simulink model "SimModel_R2019a_RL"  (R2019a)
settings: Solver=ode5  StartTime=0.0  StopTime=120  FixedStep=dt  RelTol=1e-3  EnableMultiTasking=on
values from neighbouring files (symbols this model uses):
  D_a1 = 0.1000    (= 0.1)    [SimModel_R2019a_RL_Para.m]
  D_a2 = 0.0500    (= 0.05)    [SimModel_R2019a_RL_Para.m]
  D_a3 = 3.7000    (= 3.7)    [SimModel_R2019a_RL_Para.m]
  D_a4 = 0.0    (= 0)    [SimModel_R2019a_RL_Para.m]
  D_K2 = 1.0*1.00    (= 1)    [SimModel_R2019a_RL_Para.m]
  D_Knms = 1.0    (= 1)    [SimModel_R2019a_RL_Para.m]
  D_TFar = 1.0    (= 1)    [SimModel_R2019a_RL_Para.m]
  D_Tn = 0.1000    (= 0.1)    [SimModel_R2019a_RL_Para.m]
  D_TNear = 0.3    [SimModel_R2019a_RL_Para.m]
  Et = 0.026    [SimModel_R2019a_RL_Para.m]
  Gain_EA_Far = 0    [SimModel_R2019a_RL_Para.m]
  H_a1 = 2.000    (= 2)    [SimModel_R2019a_RL_Para.m]
  H_a2 = 0.0500    (= 0.05)    [SimModel_R2019a_RL_Para.m]
  H_a3 = 40.0    (= 40)    [SimModel_R2019a_RL_Para.m]
  H_a4 = 1.0    (= 1)    [SimModel_R2019a_RL_Para.m]
  H_TFar = 0.7    [SimModel_R2019a_RL_Para.m]
  H_TNear = 0.3    [SimModel_R2019a_RL_Para.m]
  I = 300*9.8    (= 2940)    [SimModel_R2019a_RL_Para.m]
  Ih = 0.11    [SimModel_R2019a_RL_Para.m]
  K1 = 1    [SimModel_R2019a_RL_Para.m]
  Kda = 0.57    [SimModel_R2019a_RL_Para.m]
  Kf = 5.33e+04    (= 53300)    [SimModel_R2019a_RL_Para.m]
  Kr = 1.17e+05    (= 117000)    [SimModel_R2019a_RL_Para.m]
  Ks = 4950*9.8    (= 48510)    [SimModel_R2019a_RL_Para.m]
  Ksa = 0.0    (= 0)    [SimModel_R2019a_RL_Para.m]
  Kt = 1/17    (= 0.0588235294118)    [SimModel_R2019a_RL_Para.m]
  lf = 1.00    (= 1)    [SimModel_R2019a_RL_Para.m]
  lr = 1.635    [SimModel_R2019a_RL_Para.m]
  m = 1100    [SimModel_R2019a_RL_Para.m]
  TT = csvread('XY_TT.csv',0,1)    [SimModel_R2019a_RL_Para.m]
  V = 60/3.6    (= 16.6666666667)    [SimModel_R2019a_RL_Para.m]
undefined symbols (not defined in the file or in its folder): Band_TH, D_KHG, D_Kw, D_Td, dt, H_K2, Random_Disturbance
libraries: simulink x3, rllib x1
settings Model: ModifiedByFormat=kelejichi  Creator=kelejichi  LastModifiedBy=kelejichi
settings DataIOCC: SaveFormat=Array  SignalLoggingSaveFormat=ModelDataLogs
settings OptimizationCC: ExpressionDepthLimit=2147483647  InitFltsAndDblsToZero=on  LifeSpan=inf
settings DebuggingCC: UnderspecifiedInitializationDetection=Classic  MergeDetectMultiDrivingBlocksExec=none  SolverPrmCheckMsg=warning  FcnCallInpInsideContextMsg=warning  AllowSymbolicDim=off  StateNameClashWarn=warning  SFUnexpectedBacktrackingDiag=warning  SFNoUnconditionalDefaultTransitionDiag=warning  SFExecutionAtInitializationDiag=none  ArithmeticOperatorsInVariantConditions=warning
settings HardwareCC: ProdBitPerPointer=32  ProdBitPerSizeT=32  ProdBitPerPtrDiffT=32  ProdLargestAtomicFloat=None  ProdIntDivRoundTo=Undefined  ProdEndianess=Unspecified  ProdWordSize=32  ProdHWDeviceType=32-bit Generic
settings ModelReferenceCC: PropagateSignalLabelsOutOfModel=off
settings SFSimCC: SimUseLocalCustomCode=off
settings RTWCC: RTWUseLocalCustomCode=off
settings CodeAppCC: StateflowObjectComments=on
settings GRTTargetCC: TargetLangStandard=C89/C90 (ANSI)  GeneratePreprocessorConditionals=Disable all  CombineOutputUpdateFcns=off  GRTInterface=on
settings ConfigComp: CovMetricSettings=dw  CovHtmlReporting=on  CovSaveCumulativeToWorkspaceVar=on  CovSaveSingleToWorkspaceVar=on  CovExternalEMLEnable=off

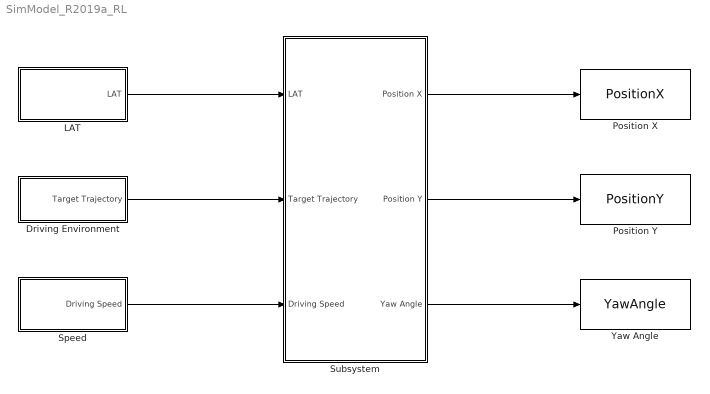
== system SimModel_R2019a_RL ==
  Driving Environment : Subsystem
  LAT : Subsystem
  Position X : ToWorkspace  VariableName=PositionX  SaveFormat=Timeseries  SampleTime=-1
  Position Y : ToWorkspace  VariableName=PositionY  SaveFormat=Timeseries  SampleTime=-1
  Speed : Subsystem
  Subsystem : Subsystem
  Yaw Angle : ToWorkspace  VariableName=YawAngle  SaveFormat=Timeseries  SampleTime=-1
  wires:
  Speed/1(Driving Speed) -> Subsystem/3(Driving Speed)
  Driving Environment/1(Target Trajectory) -> Subsystem/2(Target Trajectory)
  Subsystem/1(Position X) -> Position X/1
  Subsystem/2(Position Y) -> Position Y/1
  Subsystem/3(Yaw Angle) -> Yaw Angle/1
  LAT/1(LAT) -> Subsystem/1(LAT)

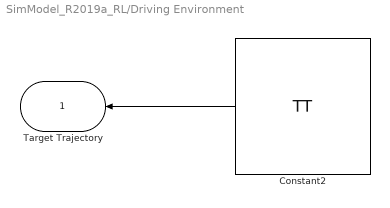
== system SimModel_R2019a_RL/Driving Environment ==
  Constant2 : Constant  Value=TT
  Target Trajectory : Outport
  wires:
  Constant2/1 -> Target Trajectory/1

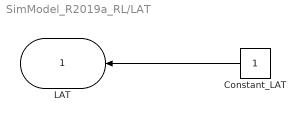
== system SimModel_R2019a_RL/LAT ==
  Constant_LAT : Constant
  LAT : Outport
  wires:
  Constant_LAT/1 -> LAT/1

== system SimModel_R2019a_RL/Speed ==
  Constant1 : Constant  Value=V
  Driving Speed : Outport
  wires:
  Constant1/1 -> Driving Speed/1

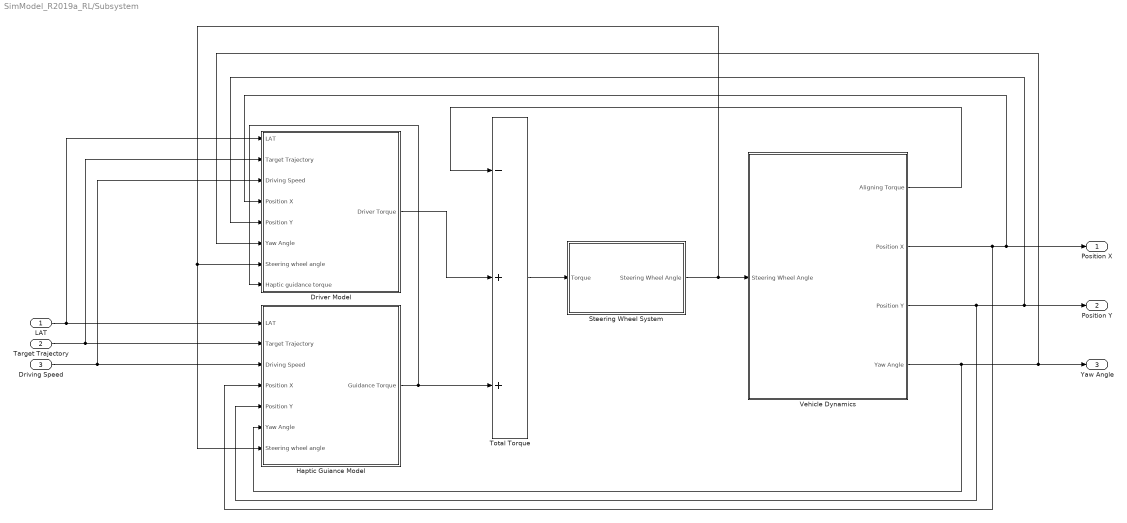
== system SimModel_R2019a_RL/Subsystem ==
  LAT : Inport
  Target Trajectory : Inport  Port=2
  Driving Speed : Inport  Port=3
  Driver Model : Subsystem
  Haptic Guiance Model : Subsystem
  Steering Wheel System : Subsystem
  Total Torque : Sum  Inputs=-++
  Vehicle Dynamics : Subsystem
  Position X : Outport
  Position Y : Outport  Port=2
  Yaw Angle : Outport  Port=3
  wires:
  Vehicle Dynamics/1(Aligning Torque) -> Total Torque/1
  Vehicle Dynamics/2(Position X) -> Position X/1, Driver Model/4(Position X), Haptic Guiance Model/4(Position X)
  Total Torque/1 -> Steering Wheel System/1(Torque)
  Driving Speed/1 -> Haptic Guiance Model/3(Driving Speed), Driver Model/3(Driving Speed)
  Target Trajectory/1 -> Driver Model/2(Target Trajectory), Haptic Guiance Model/2(Target Trajectory)
  Haptic Guiance Model/1(Guidance Torque) -> Total Torque/3, Driver Model/8(Haptic guidance torque)
  Vehicle Dynamics/3(Position Y) -> Position Y/1, Driver Model/5(Position Y), Haptic Guiance Model/5(Position Y)
  Vehicle Dynamics/4(Yaw Angle) -> Yaw Angle/1, Driver Model/6(Yaw Angle), Haptic Guiance Model/6(Yaw Angle)
  Driver Model/1(Driver Torque) -> Total Torque/2
  LAT/1 -> Driver Model/1(LAT), Haptic Guiance Model/1(LAT)
  Steering Wheel System/1(Steering Wheel Angle) -> Driver Model/7(Steering wheel angle), Haptic Guiance Model/7(Steering wheel angle), Vehicle Dynamics/1(Steering Wheel Angle)

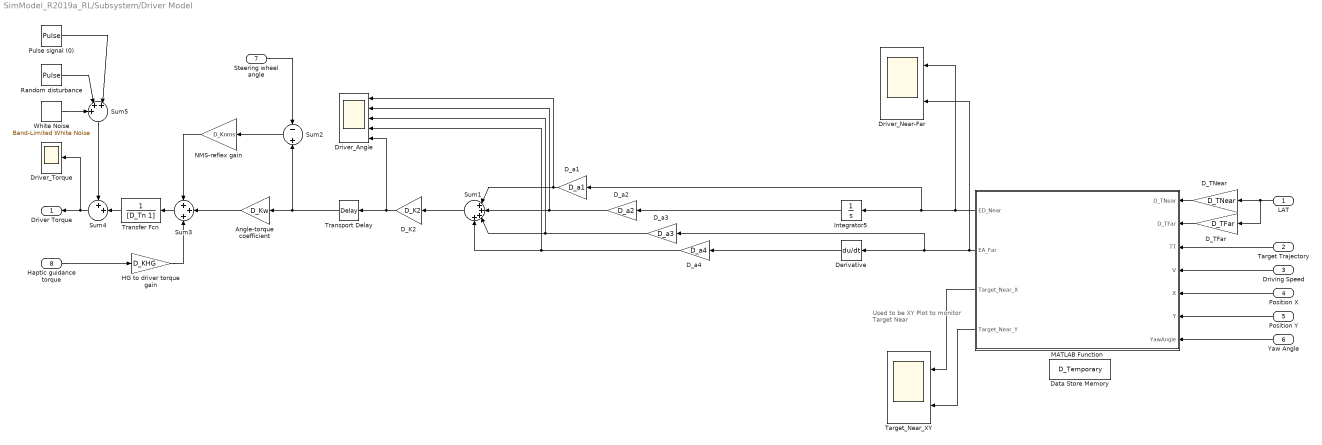
== system SimModel_R2019a_RL/Subsystem/Driver Model ==
  note: Used to be XY Plot to monitor Target Near
  LAT : Inport
  Target Trajectory : Inport  Port=2
  Driving Speed : Inport  Port=3
  Position X : Inport  Port=4
  Position Y : Inport  Port=5
  Yaw Angle : Inport  Port=6
  Steering wheel angle : Inport  Port=7
  Haptic guidance torque : Inport  Port=8
  Angle-torque coefficient : Gain  Gain=D_Kw
  D_K2 : Gain  Gain=D_K2
  D_TFar : Gain  Gain=D_TFar
  D_TNear : Gain  Gain=D_TNear
  D_a1 : Gain  Gain=D_a1
  D_a2 : Gain  Gain=D_a2
  D_a3 : Gain  Gain=D_a3
  D_a4 : Gain  Gain=D_a4
  Data Store Memory : DataStoreMemory  DataStoreName=D_Temporary  ReadBeforeWriteMsg=warning  WriteAfterWriteMsg=warning  WriteAfterReadMsg=warning  InitialValue=2  ShowAdditionalParam=off  OutDataTypeStr=double
  Derivative : Derivative
  Driver_Angle : Scope  NumInputPorts=5
  Driver_Near-Far : Scope  NumInputPorts=2
  Driver_Torque : Scope
  HG to driver torque gain : Gain  Gain=D_KHG
  Integrator5 : Integrator
  MATLAB Function : MATLAB Function  TreatAsAtomicUnit=on
  NMS-reflex gain : Gain  Gain=D_Knms
  Pulse signal (0) : DiscretePulseGenerator  PulseType=Time based  Amplitude=0  Period=20  PulseWidth=10  PhaseDelay=32
  Random disturbance : DiscretePulseGenerator  PulseType=Time based  Amplitude=0.1  Period=20  PulseWidth=10  PhaseDelay=Random_Disturbance
  Sum1 : Sum  Inputs=|++++
  Sum2 : Sum  Inputs=-+
  Sum3 : Sum  Inputs=+++
  Sum4 : Sum  Inputs=++|
  Sum5 : Sum  Inputs=+++|
  Target_Near_XY : Scope  NumInputPorts=2
  Transfer Fcn : TransferFcn  Denominator=[D_Tn 1]
  Transport Delay : TransportDelay  DelayTime=D_Td
  White Noise : simulink/Sources/Band-Limited White Noise  Cov=D_WN  Ts=dt  seed=[23341]
  Driver Torque : Outport
  wires:
  MATLAB Function/1(ED_Near) -> Driver_Near-Far/1, D_a1/1, Integrator5/1
  Integrator5/1 -> D_a2/1
  MATLAB Function/2(EA_Far) -> Driver_Near-Far/2, D_a3/1, Derivative/1
  Derivative/1 -> D_a4/1
  Target Trajectory/1 -> MATLAB Function/3(TT)
  Position X/1 -> MATLAB Function/5(X)
  Position Y/1 -> MATLAB Function/6(Y)
  Yaw Angle/1 -> MATLAB Function/7(YawAngle)
  Driving Speed/1 -> MATLAB Function/4(V)
  D_a1/1 -> Driver_Angle/1, Sum1/1
  D_a2/1 -> Driver_Angle/2, Sum1/2
  D_a3/1 -> Driver_Angle/3, Sum1/3
  D_a4/1 -> Driver_Angle/4, Sum1/4
  Sum1/1 -> D_K2/1
  D_K2/1 -> Driver_Angle/5, Transport Delay/1
  Transport Delay/1 -> Angle-torque coefficient/1, Sum2/2
  Sum4/1 -> Driver_Torque/1, Driver Torque/1
  LAT/1 -> D_TFar/1, D_TNear/1
  D_TNear/1 -> MATLAB Function/1(D_TNear)
  D_TFar/1 -> MATLAB Function/2(D_TFar)
  Angle-torque coefficient/1 -> Sum3/2
  Sum3/1 -> Transfer Fcn/1
  NMS-reflex gain/1 -> Sum3/1
  Sum2/1 -> NMS-reflex gain/1
  Steering wheel angle/1 -> Sum2/1
  HG to driver torque gain/1 -> Sum3/3
  Haptic guidance torque/1 -> HG to driver torque gain/1
  Transfer Fcn/1 -> Sum4/2
  Random disturbance/1 -> Sum5/2
  White Noise/1 -> Sum5/1
  Sum5/1 -> Sum4/1
  Pulse signal (0)/1 -> Sum5/3
  MATLAB Function/3(Target_Near_X) -> Target_Near_XY/1
  MATLAB Function/4(Target_Near_Y) -> Target_Near_XY/2

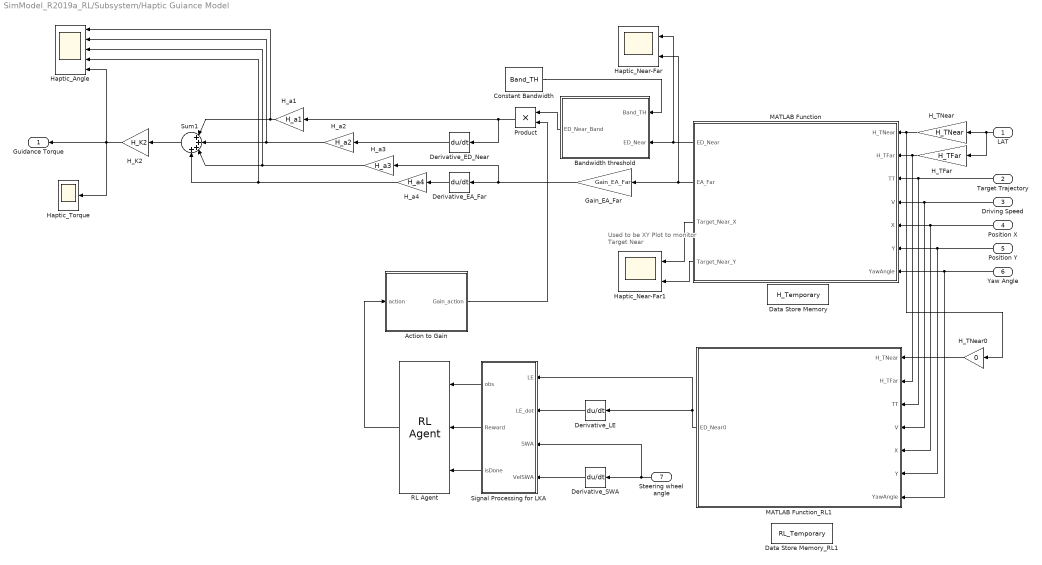
== system SimModel_R2019a_RL/Subsystem/Haptic Guiance Model ==
  note: Used to be XY Plot to monitor Target Near
  LAT : Inport
  Target Trajectory : Inport  Port=2
  Driving Speed : Inport  Port=3
  Position X : Inport  Port=4
  Position Y : Inport  Port=5
  Yaw Angle : Inport  Port=6
  Steering wheel angle : Inport  Port=7
  Action to Gain : MATLAB Function  TreatAsAtomicUnit=on
  Bandwidth threshold : MATLAB Function  TreatAsAtomicUnit=on
  Constant Bandwidth : Constant  Value=Band_TH
  Data Store Memory : DataStoreMemory  DataStoreName=H_Temporary  ReadBeforeWriteMsg=warning  WriteAfterWriteMsg=warning  WriteAfterReadMsg=warning  InitialValue=2  ShowAdditionalParam=off  OutDataTypeStr=double
  "Data Store Memory_RL1 " : DataStoreMemory  DataStoreName=RL_Temporary  ReadBeforeWriteMsg=warning  WriteAfterWriteMsg=warning  WriteAfterReadMsg=warning  InitialValue=2  ShowAdditionalParam=off  OutDataTypeStr=double
  Derivative_EA_Far : Derivative
  Derivative_ED_Near : Derivative
  Derivative_LE : Derivative
  Derivative_SWA : Derivative
  Gain_EA_Far : Gain  Gain=Gain_EA_Far
  H_K2 : Gain  Gain=H_K2
  H_TFar : Gain  Gain=H_TFar
  H_TNear : Gain  Gain=H_TNear
  H_TNear0 : Gain  Gain=0
  H_a1 : Gain  Gain=H_a1
  H_a2 : Gain  Gain=H_a2
  H_a3 : Gain  Gain=H_a3
  H_a4 : Gain  Gain=H_a4
  Haptic_Angle : Scope  NumInputPorts=5
  Haptic_Near-Far : Scope  NumInputPorts=2
  Haptic_Near-Far1 : Scope  NumInputPorts=2
  Haptic_Torque : Scope
  MATLAB Function : MATLAB Function  TreatAsAtomicUnit=on
  MATLAB Function_RL1 : MATLAB Function  TreatAsAtomicUnit=on
  Product : Product
  RL Agent : rllib/RL Agent  Agent=agent  ProvideReward=on  ProvideIsDone=on  ProvideCumRwd=off  TreatAsDirectFeedthrough=on  CollectLoggedSignals=on  CollectModelStates=on
      settings: SourceProductName=Reinforcement Learning Toolbox
  "Signal Processing for LKA " : Subsystem
  Sum1 : Sum  Inputs=|++++
  Guidance Torque : Outport
  wires:
  MATLAB Function/1(ED_Near) -> Haptic_Near-Far/1, Bandwidth threshold/2(ED_Near)
  Derivative_ED_Near/1 -> H_a2/1
  MATLAB Function/2(EA_Far) -> Haptic_Near-Far/2, Gain_EA_Far/1
  Derivative_EA_Far/1 -> H_a4/1
  Target Trajectory/1 -> MATLAB Function_RL1/3(TT), MATLAB Function/3(TT)
  Position X/1 -> MATLAB Function_RL1/5(X), MATLAB Function/5(X)
  Position Y/1 -> MATLAB Function_RL1/6(Y), MATLAB Function/6(Y)
  Yaw Angle/1 -> MATLAB Function_RL1/7(YawAngle), MATLAB Function/7(YawAngle)
  Driving Speed/1 -> MATLAB Function_RL1/4(V), MATLAB Function/4(V)
  H_a1/1 -> Haptic_Angle/1, Sum1/1
  H_a2/1 -> Haptic_Angle/2, Sum1/2
  H_a3/1 -> Haptic_Angle/3, Sum1/3
  H_a4/1 -> Haptic_Angle/4, Sum1/4
  Sum1/1 -> H_K2/1
  H_K2/1 -> Haptic_Torque/1, Haptic_Angle/5, Guidance Torque/1
  LAT/1 -> H_TFar/1, H_TNear/1
  H_TNear/1 -> H_TNear0/1, MATLAB Function/1(H_TNear)
  H_TFar/1 -> MATLAB Function_RL1/2(H_TFar), MATLAB Function/2(H_TFar)
  Product/1 -> Derivative_ED_Near/1, H_a1/1
  Gain_EA_Far/1 -> H_a3/1, Derivative_EA_Far/1
  H_TNear0/1 -> MATLAB Function_RL1/1(H_TNear)
  RL Agent/1 -> Action to Gain/1(action)
  Constant Bandwidth/1 -> Bandwidth threshold/1(Band_TH)
  Bandwidth threshold/1(ED_Near_Band) -> Product/1
  Action to Gain/1(Gain_action) -> Product/2
  "Signal Processing for LKA "/1(obs) -> RL Agent/1
  "Signal Processing for LKA "/2(Reward) -> RL Agent/2
  "Signal Processing for LKA "/3(isDone) -> RL Agent/3
  Derivative_SWA/1 -> "Signal Processing for LKA "/4("VelSWA ")
  Steering wheel angle/1 -> "Signal Processing for LKA "/3(SWA), Derivative_SWA/1
  MATLAB Function_RL1/1(ED_Near0) -> Derivative_LE/1, "Signal Processing for LKA "/1(LE)
  Derivative_LE/1 -> "Signal Processing for LKA "/2(LE_dot)
  MATLAB Function/3(Target_Near_X) -> Haptic_Near-Far1/1
  MATLAB Function/4(Target_Near_Y) -> Haptic_Near-Far1/2

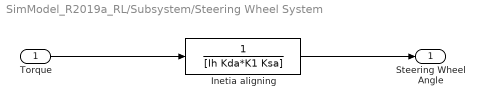
== system SimModel_R2019a_RL/Subsystem/Steering Wheel System ==
  Torque : Inport
  Inetia aligning : TransferFcn  Denominator=[Ih Kda*K1 Ksa]
  Steering Wheel Angle : Outport
  wires:
  Torque/1 -> Inetia aligning/1
  Inetia aligning/1 -> Steering Wheel Angle/1

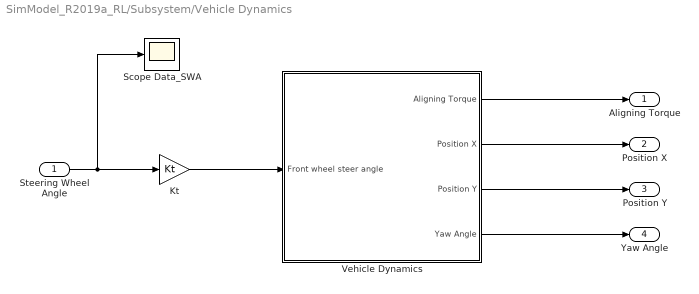
== system SimModel_R2019a_RL/Subsystem/Vehicle Dynamics ==
  Steering Wheel Angle : Inport
  Kt : Gain  Gain=Kt
  Scope Data_SWA : Scope
  Vehicle Dynamics : Subsystem
  Aligning Torque : Outport
  Position X : Outport  Port=2
  Position Y : Outport  Port=3
  Yaw Angle : Outport  Port=4
  wires:
  Vehicle Dynamics/1(Aligning Torque) -> Aligning Torque/1
  Kt/1 -> Vehicle Dynamics/1(Front wheel steer angle)
  Vehicle Dynamics/2(Position X) -> Position X/1
  Vehicle Dynamics/3(Position Y) -> Position Y/1
  Vehicle Dynamics/4(Yaw Angle) -> Yaw Angle/1
  Steering Wheel Angle/1 -> Scope Data_SWA/1, Kt/1

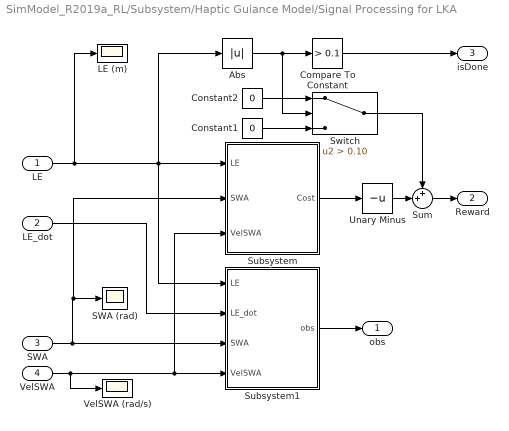
== system SimModel_R2019a_RL/Subsystem/Haptic Guiance Model/Signal Processing for LKA  ==
  LE : Inport
  LE_dot : Inport  Port=2
  SWA : Inport  Port=3
  "VelSWA " : Inport  Port=4
  Abs : Abs
  Compare To Constant : simulink/Logic and Bit Operations/Compare To Constant  relop=>  const=0.1  OutDataTypeStr=boolean
  Constant1 : Constant  Value=0
  Constant2 : Constant  Value=0
  LE (m) : Scope
  SWA (rad) : Scope
  Subsystem : Subsystem
  Subsystem1 : Subsystem
  Sum : Sum  Inputs=++|
  Switch : Switch  Criteria=u2 > Threshold  Threshold=0.10
  Unary Minus : UnaryMinus
  "VelSWA (rad/s) " : Scope
  obs : Outport
  Reward : Outport  Port=2
  isDone : Outport  Port=3
  wires:
  Subsystem/1(Cost) -> Unary Minus/1
  LE/1 -> Subsystem1/1(LE), Abs/1, Subsystem/1(LE), LE (m)/1
  SWA/1 -> Subsystem/2(SWA), SWA (rad)/1, Subsystem1/3(SWA)
  Abs/1 -> Switch/2, Compare To Constant/1
  Compare To Constant/1 -> isDone/1
  Subsystem1/1(obs) -> obs/1
  "VelSWA "/1 -> Subsystem/3(VelSWA), Subsystem1/4(VelSWA), "VelSWA (rad/s) "/1
  LE_dot/1 -> Subsystem1/2(LE_dot)
  Unary Minus/1 -> Sum/2
  Sum/1 -> Reward/1
  Constant1/1 -> Switch/3
  Switch/1 -> Sum/1
  Constant2/1 -> Switch/1

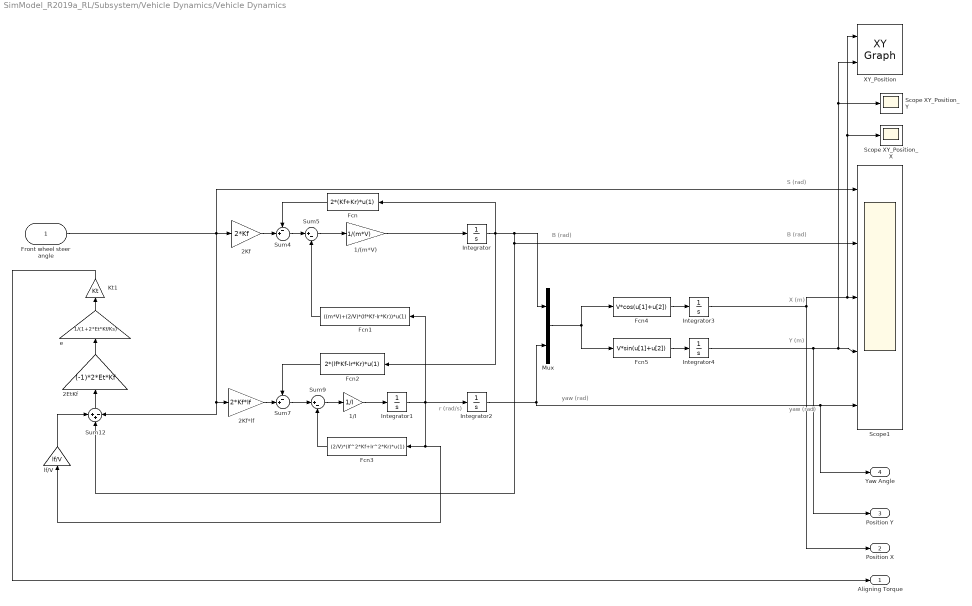
== system SimModel_R2019a_RL/Subsystem/Vehicle Dynamics/Vehicle Dynamics ==
  note: Y (m)
  note: yaw (rad)
  note: r (rad/s)
  note: S (rad)
  note: B (rad)
  note: X (m)
  note: B (rad)
  note: yaw (rad)
  Front wheel steer angle : Inport
  1/(m*V) : Gain  Gain=1/(m*V)
  1/I : Gain  Gain=1/I
  2EtKf : Gain  Gain=(-1)*2*Et*Kf
  2Kf : Gain  Gain=2*Kf
  2Kf*lf : Gain  Gain=2*Kf*lf
  Fcn : Fcn  Expr=2*(Kf+Kr)*u(1)
  Fcn1 : Fcn  Expr=((m*V)+(2/V)*(lf*Kf-lr*Kr))*u(1)
  Fcn2 : Fcn  Expr=2*(lf*Kf-lr*Kr)*u(1)
  Fcn3 : Fcn  Expr=(2/V)*(lf^2*Kf+lr^2*Kr)*u(1)
  Fcn4 : Fcn  Expr=V*cos(u[1]+u[2])
  Fcn5 : Fcn  Expr=V*sin(u[1]+u[2])
  Integrator{,1..4} (5 alike) : Integrator
  Kt1 : Gain  Gain=Kt
  Mux : Mux  Inputs=2
  Scope XY_Position_X : Scope
  Scope XY_Position_Y : Scope
  Scope1 : Scope  NumInputPorts=5
  Sum12 : Sum  Inputs=++-
  Sum4 : Sum  Inputs=-+|
  Sum5 : Sum  Inputs=|+-
  Sum7 : Sum  Inputs=-+|
  Sum9 : Sum  Inputs=|+-
  XY_Position : simulink/Sinks/XY Graph  xmin=0  xmax=7000  ymin=-5  ymax=3000  st=-1
  e : Gain  Gain=1/(1+2*Et*Kf/Ks)
  lf/V : Gain  Gain=lf/V
  Aligning Torque : Outport
  Position X : Outport  Port=2
  Position Y : Outport  Port=3
  Yaw Angle : Outport  Port=4
  wires:
  Kt1/1 -> Aligning Torque/1
  Sum12/1 -> 2EtKf/1
  Sum4/1 -> Sum5/1
  Fcn3/1 -> Sum9/2
  Fcn1/1 -> Sum5/2
  2EtKf/1 -> e/1
  1/I/1 -> Integrator1/1
  Integrator1/1 -> lf/V/1, Fcn3/1, Fcn1/1, Integrator2/1
  Sum5/1 -> 1/(m*V)/1
  Mux/1 -> Fcn5/1, Fcn4/1
  2Kf*lf/1 -> Sum7/2
  lf/V/1 -> Sum12/1
  Integrator3/1 -> XY_Position/1, Scope XY_Position_X/1, Scope1/3, Position X/1
  Fcn4/1 -> Integrator3/1
  Sum7/1 -> Sum9/1
  Integrator/1 -> Sum12/2, Scope1/2, Mux/1, Fcn/1, Fcn2/1
  1/(m*V)/1 -> Integrator/1
  Fcn5/1 -> Integrator4/1
  Sum9/1 -> 1/I/1
  Fcn2/1 -> Sum7/1
  Integrator2/1 -> Yaw Angle/1, Scope1/5, Mux/2
  Fcn/1 -> Sum4/1
  2Kf/1 -> Sum4/2
  Integrator4/1 -> Position Y/1, Scope XY_Position_Y/1, XY_Position/2, Scope1/4
  Front wheel steer angle/1 -> Scope1/1, 2Kf*lf/1, Sum12/3, 2Kf/1
  e/1 -> Kt1/1

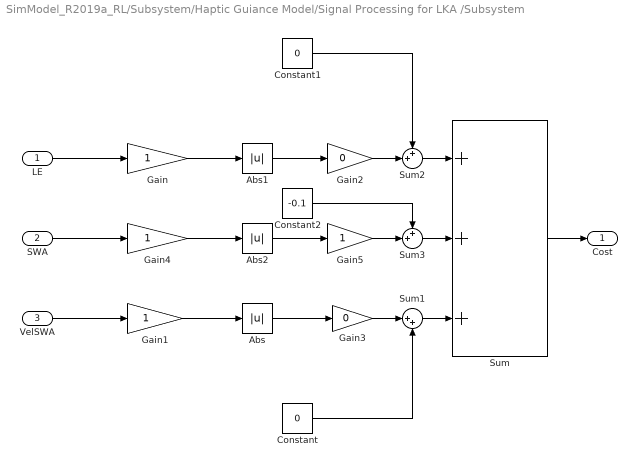
== system SimModel_R2019a_RL/Subsystem/Haptic Guiance Model/Signal Processing for LKA /Subsystem ==
  LE : Inport
  SWA : Inport  Port=2
  VelSWA : Inport  Port=3
  Abs : Abs
  Abs1 : Abs
  Abs2 : Abs
  Constant : Constant  Value=0
  Constant1 : Constant  Value=0
  Constant2 : Constant  Value=-0.1
  Gain{,1,4..5} (4 alike) : Gain
  Gain2 : Gain  Gain=0
  Gain3 : Gain  Gain=0
  Sum : Sum  Inputs=+++
  Sum1 : Sum  Inputs=|++
  Sum2 : Sum  Inputs=++|
  Sum3 : Sum  Inputs=++|
  Cost : Outport
  wires:
  LE/1 -> Gain/1
  VelSWA/1 -> Gain1/1
  Sum/1 -> Cost/1
  Abs1/1 -> Gain2/1
  Gain1/1 -> Abs/1
  Gain/1 -> Abs1/1
  Gain3/1 -> Sum1/1
  Abs/1 -> Gain3/1
  Constant/1 -> Sum1/2
  Sum1/1 -> Sum/3
  Sum2/1 -> Sum/1
  Gain2/1 -> Sum2/2
  Constant1/1 -> Sum2/1
  Constant2/1 -> Sum3/1
  Gain4/1 -> Abs2/1
  Gain5/1 -> Sum3/2
  SWA/1 -> Gain4/1
  Abs2/1 -> Gain5/1
  Sum3/1 -> Sum/2

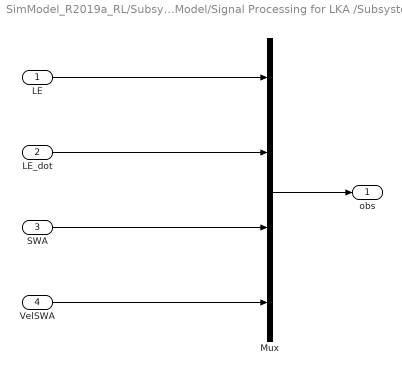
== system SimModel_R2019a_RL/Subsystem/Haptic Guiance Model/Signal Processing for LKA /Subsystem1 ==
  LE : Inport
  LE_dot : Inport  Port=2
  SWA : Inport  Port=3
  VelSWA : Inport  Port=4
  Mux : Mux
  obs : Outport
  wires:
  LE/1 -> Mux/1
  Mux/1 -> obs/1
  SWA/1 -> Mux/3
  VelSWA/1 -> Mux/4
  LE_dot/1 -> Mux/2

== matlab function SimModel_R2019a_RL/Subsystem/Driver Model/MATLAB Function ==
  settings: updateMethod=DISCRETE  sampleTime=dt
  data: D_TNear input; D_TFar input; TT input; V input; X input; ED_Near output; Y input; YawAngle input; EA_Far output; Target_Near_X output; Target_Near_Y output; D_Temporary data_store_memory
function [ED_Near,EA_Far,Target_Near_X,Target_Near_Y] = fcn(D_TNear,D_TFar,TT,V,X,Y,YawAngle)
%#codegen
%% Global variable
global D_Temporary;
%% Setting
% Data Input
dfw_Xv = X;
dfw_Yv = Y;
dff_Psivdb = YawAngle;
% Parameters
Range_XY = 100;
sRun_entire = TT;
Spd = V;
LAT_Near = D_TNear;
LAT_Far  = D_TFar;
% Look ahead point
LAP_Near_X  = dfw_Xv + Spd * LAT_Near * cos(dff_Psivdb);
LAP_Near_Y  = dfw_Yv + Spd * LAT_Near * sin(dff_Psivdb);
LAP_Near_XY = [LAP_Near_X,LAP_Near_Y];
LAP_Far_X   = dfw_Xv + Spd * LAT_Far  * cos(dff_Psivdb);
LAP_Far_Y   = dfw_Yv + Spd * LAT_Far  * sin(dff_Psivdb);
LAP_Far_XY  = [LAP_Far_X,LAP_Far_Y];
% %% Find the proper range of target trajectory to reduce the calculation time
% for i_Range = 1:(length(sRun_entire)-1)
%     sRun_start = i_Range;
%     if norm((dfw_Xv-sRun_entire(i_Range,1)),(dfw_Yv-sRun_entire(i_Range,2))) < Range_XY
%                 break;
%     end
% end
% sRun = sRun_entire(sRun_start:(sRun_start+Range_XY*100),:); 
%% Start from Temporary-1
sRun_start = D_Temporary-1;
sRun = sRun_entire(sRun_start:(sRun_start+Range_XY*30/2),:); 
%% Error Calculation (dx,dy,n1x,n1y,n2x,n2y:dot(a,b)*dot(a,c)<=0)
% Near Point
for i_Near = 1:(length(sRun)-2)
    Vec_Near_a1 = sRun(i_Near+1,:) - sRun(i_Near,:);
    Vec_Near_b1 = LAP_Near_XY - sRun(i_Near,:);
    Vec_Near_c1 = LAP_Near_XY - sRun(i_Near+1,:);
    Vec_Near_a2 = sRun(i_Near+2,:) - sRun(i_Near+1,:);
    Vec_Near_b2 = LAP_Near_XY - sRun(i_Near+1,:);
    Vec_Near_c2 = LAP_Near_XY - sRun(i_Near+2,:);
    if (dot(Vec_Near_a1,Vec_Near_b1) * dot(Vec_Near_a2,Vec_Near_c2)) <= 0
        break;
    end

end

Target_Near = sRun(i_Near,:);
Target_Near_X = sRun(i_Near,1);
Target_Near_Y = sRun(i_Near,2);

ED_Near = norm(Vec_Near_b1) * sin(atan2(Vec_Near_a1(1,2),Vec_Near_a1(1,1))-atan2(Vec_Near_b1(1,2),Vec_Near_b1(1,1)));

% Far Point
for i_Far = 1:(length(sRun)-2)
    Vec_Far_a1 = sRun(i_Far+1,:) - sRun(i_Far,:);
    Vec_Far_b1 = LAP_Far_XY - sRun(i_Far,:);
    Vec_Far_c1 = LAP_Far_XY - sRun(i_Far+1,:);
    Vec_Far_a2 = sRun(i_Far+2,:) - sRun(i_Far+1,:);
    Vec_Far_b2 = LAP_Far_XY - sRun(i_Far+1,:);
    Vec_Far_c2 = LAP_Far_XY - sRun(i_Far+2,:);
    if (dot(Vec_Far_a1,Vec_Far_b1) * dot(Vec_Far_a2,Vec_Far_c2)) <= 0
        break;
    end
end
Target_Far = sRun(i_Far,:);
Target_Far_X = sRun(i_Far,1);
Target_Far_Y = sRun(i_Far,2);

EA_Far = atan2(Vec_Far_a1(1,2),Vec_Far_a1(1,1))-dff_Psivdb;
%% Temporary
D_Temporary = i_Near + sRun_start;

== matlab function SimModel_R2019a_RL/Subsystem/Haptic Guiance Model/MATLAB Function ==
  settings: updateMethod=DISCRETE  sampleTime=dt
  data: H_TNear input; H_TFar input; TT input; V input; X input; ED_Near output; Y input; YawAngle input; EA_Far output; Target_Near_X output; Target_Near_Y output; H_Temporary data_store_memory
function [ED_Near,EA_Far,Target_Near_X,Target_Near_Y] = fcn(H_TNear,H_TFar,TT,V,X,Y,YawAngle)
%#codegen
%% Global variable
global H_Temporary;
%% Setting
% Data Input
dfw_Xv = X;
dfw_Yv = Y;
dff_Psivdb = YawAngle;
% Parameters
Range_XY = 100;
sRun_entire = TT;
Spd = V;
LAT_Near = H_TNear;
LAT_Far  = H_TFar;
% Look ahead point
LAP_Near_X  = dfw_Xv + Spd * LAT_Near * cos(dff_Psivdb);
LAP_Near_Y  = dfw_Yv + Spd * LAT_Near * sin(dff_Psivdb);
LAP_Near_XY = [LAP_Near_X,LAP_Near_Y];
LAP_Far_X   = dfw_Xv + Spd * LAT_Far  * cos(dff_Psivdb);
LAP_Far_Y   = dfw_Yv + Spd * LAT_Far  * sin(dff_Psivdb);
LAP_Far_XY  = [LAP_Far_X,LAP_Far_Y];
% %% Find the proper range of target trajectory to reduce the calculation time
% for i_Range = 1:(length(sRun_entire)-1)
%     sRun_start = i_Range;
%     if norm((dfw_Xv-sRun_entire(i_Range,1)),(dfw_Yv-sRun_entire(i_Range,2))) < Range_XY
%                 break;
%     end
% end
% sRun = sRun_entire(sRun_start:(sRun_start+Range_XY*100),:);   
%% Start from Temporary-1
sRun_start = H_Temporary-1;
sRun = sRun_entire(sRun_start:(sRun_start+Range_XY*30/2),:); 
%% Error Calculation (dx,dy,n1x,n1y,n2x,n2y:dot(a,b)*dot(a,c)<=0)
% Near Point
for i_Near = 1:(length(sRun)-2)
    Vec_Near_a1 = sRun(i_Near+1,:) - sRun(i_Near,:);
    Vec_Near_b1 = LAP_Near_XY - sRun(i_Near,:);
    Vec_Near_c1 = LAP_Near_XY - sRun(i_Near+1,:);
    Vec_Near_a2 = sRun(i_Near+2,:) - sRun(i_Near+1,:);
    Vec_Near_b2 = LAP_Near_XY - sRun(i_Near+1,:);
    Vec_Near_c2 = LAP_Near_XY - sRun(i_Near+2,:);
    if (dot(Vec_Near_a1,Vec_Near_b1) * dot(Vec_Near_a2,Vec_Near_c2)) <= 0
        break;
    end

end

Target_Near = sRun(i_Near,:);
Target_Near_X = sRun(i_Near,1);
Target_Near_Y = sRun(i_Near,2);

ED_Near = norm(Vec_Near_b1) * sin(atan2(Vec_Near_a1(1,2),Vec_Near_a1(1,1))-atan2(Vec_Near_b1(1,2),Vec_Near_b1(1,1)));

% Far Point
for i_Far = 1:(length(sRun)-2)
    Vec_Far_a1 = sRun(i_Far+1,:) - sRun(i_Far,:);
    Vec_Far_b1 = LAP_Far_XY - sRun(i_Far,:);
    Vec_Far_c1 = LAP_Far_XY - sRun(i_Far+1,:);
    Vec_Far_a2 = sRun(i_Far+2,:) - sRun(i_Far+1,:);
    Vec_Far_b2 = LAP_Far_XY - sRun(i_Far+1,:);
    Vec_Far_c2 = LAP_Far_XY - sRun(i_Far+2,:);
    if (dot(Vec_Far_a1,Vec_Far_b1) * dot(Vec_Far_a2,Vec_Far_c2)) <= 0
        break;
    end
end
Target_Far = sRun(i_Far,:);
Target_Far_X = sRun(i_Far,1);
Target_Far_Y = sRun(i_Far,2);

EA_Far = atan2(Vec_Far_a1(1,2),Vec_Far_a1(1,1))-dff_Psivdb;
%% Temporary
H_Temporary = i_Near + sRun_start;

== matlab function SimModel_R2019a_RL/Subsystem/Haptic Guiance Model/Bandwidth threshold ==
  data: Band_TH input; ED_Near input; ED_Near_Band output
function ED_Near_Band = fcn(Band_TH,ED_Near)
%#codegen

if abs(ED_Near) > Band_TH 
    ED_Near_Band = ED_Near;
else
    ED_Near_Band = 0;
end

== matlab function SimModel_R2019a_RL/Subsystem/Haptic Guiance Model/MATLAB Function_RL1 ==
  settings: updateMethod=DISCRETE  sampleTime=dt
  data: H_TNear input; H_TFar input; TT input; V input; X input; ED_Near0 output; Y input; YawAngle input; RL_Temporary data_store_memory
function ED_Near0  = fcn(H_TNear,H_TFar,TT,V,X,Y,YawAngle)
%#codegen
%% Global variable
global RL_Temporary;
%% Setting
% Data Input
dfw_Xv = X;
dfw_Yv = Y;
dff_Psivdb = YawAngle;
% Parameters
Range_XY = 100;
sRun_entire = TT;
Spd = V;
LAT_Near = H_TNear;
LAT_Far  = H_TFar;
% Look ahead point
LAP_Near_X  = dfw_Xv + Spd * LAT_Near * cos(dff_Psivdb);
LAP_Near_Y  = dfw_Yv + Spd * LAT_Near * sin(dff_Psivdb);
LAP_Near_XY = [LAP_Near_X,LAP_Near_Y];
LAP_Far_X   = dfw_Xv + Spd * LAT_Far  * cos(dff_Psivdb);
LAP_Far_Y   = dfw_Yv + Spd * LAT_Far  * sin(dff_Psivdb);
LAP_Far_XY  = [LAP_Far_X,LAP_Far_Y];
% %% Find the proper range of target trajectory to reduce the calculation time
% for i_Range = 1:(length(sRun_entire)-1)
%     sRun_start = i_Range;
%     if norm((dfw_Xv-sRun_entire(i_Range,1)),(dfw_Yv-sRun_entire(i_Range,2))) < Range_XY
%                 break;
%     end
% end
% sRun = sRun_entire(sRun_start:(sRun_start+Range_XY*100),:);   
%% Start from Temporary-1
sRun_start = RL_Temporary-1;
sRun = sRun_entire(sRun_start:(sRun_start+Range_XY*30/2),:); 
%% Error Calculation (dx,dy,n1x,n1y,n2x,n2y:dot(a,b)*dot(a,c)<=0)
% Near Point
for i_Near = 1:(length(sRun)-2)
    Vec_Near_a1 = sRun(i_Near+1,:) - sRun(i_Near,:);
    Vec_Near_b1 = LAP_Near_XY - sRun(i_Near,:);
    Vec_Near_c1 = LAP_Near_XY - sRun(i_Near+1,:);
    Vec_Near_a2 = sRun(i_Near+2,:) - sRun(i_Near+1,:);
    Vec_Near_b2 = LAP_Near_XY - sRun(i_Near+1,:);
    Vec_Near_c2 = LAP_Near_XY - sRun(i_Near+2,:);
    if (dot(Vec_Near_a1,Vec_Near_b1) * dot(Vec_Near_a2,Vec_Near_c2)) <= 0
        break;
    end

end

Target_Near = sRun(i_Near,:);
Target_Near_X = sRun(i_Near,1);
Target_Near_Y = sRun(i_Near,2);

ED_Near0 = norm(Vec_Near_b1) * sin(atan2(Vec_Near_a1(1,2),Vec_Near_a1(1,1))-atan2(Vec_Near_b1(1,2),Vec_Near_b1(1,1)));

% Far Point
for i_Far = 1:(length(sRun)-2)
    Vec_Far_a1 = sRun(i_Far+1,:) - sRun(i_Far,:);
    Vec_Far_b1 = LAP_Far_XY - sRun(i_Far,:);
    Vec_Far_c1 = LAP_Far_XY - sRun(i_Far+1,:);
    Vec_Far_a2 = sRun(i_Far+2,:) - sRun(i_Far+1,:);
    Vec_Far_b2 = LAP_Far_XY - sRun(i_Far+1,:);
    Vec_Far_c2 = LAP_Far_XY - sRun(i_Far+2,:);
    if (dot(Vec_Far_a1,Vec_Far_b1) * dot(Vec_Far_a2,Vec_Far_c2)) <= 0
        break;
    end
end
Target_Far = sRun(i_Far,:);
Target_Far_X = sRun(i_Far,1);
Target_Far_Y = sRun(i_Far,2);

EA_Far = atan2(Vec_Far_a1(1,2),Vec_Far_a1(1,1))-dff_Psivdb;
%% Temporary
RL_Temporary = i_Near + sRun_start;

== matlab function SimModel_R2019a_RL/Subsystem/Haptic Guiance Model/Action to Gain ==
  data: action input; Gain_action output
function Gain_action = fcn(action)
%#codegen

Gain_action = action;


end
